simulink model "rfdc_awg"  (R2021a)
(part 2 of 30)

      mask prompts: io_names "Names [msb...lsb]"; io_widths "Bitwidths [msb...lsb]"; io_bps "Binary pts [msb...lsb]"; io_types "Data types [msb...lsb], ufix=0, fix=1, bool=2"; show_format "Print format string?"; snap_storage "Storage medium"; snap_dram_dimm "DRAM dimm"; snap_dram_clock "DRAM clock rate"; snap_nsamples "Number of Samples (2^?)"; snap_data_width "Data width"; snap_offset "Start delay support"; snap_circap "Circular capture support"; snap_value "Extra value capture support"; snap_ext_arm "External arm support"; snap_ext_circ "External circular capture support"; snap_provide_outputs "Provide outputs"; snap_use_dsp48 "Use DSP48s to implement counters"; snap_delay "Pre-snapshot delay"; extra_names "Names [msb...lsb]"; extra_widths "Widths [msb...lsb]"; extra_bps "Binary pts [msb...lsb]"; extra_types "Data types [msb...lsb], ufix=0, fix=1, bool=2"
      mask help:
      | A wrapped snapshot block. Allows specification of inputs to a snapblock word so the toolflow can automatically set up the scope.
      | See documentation for snapshot for explanation of parameters.
      mask init:
      | bitsnap_init(gcb);
      settings: AttributesFormatString=|
      | snap(1):uf128.0 = 128 bits\n128 wide, 16384 deep
      | debugID: 89627792
      mask TypeOptions snap_storage: bram | dram
      mask Callback snap_storage: bitsnap_callback();
      mask TypeOptions snap_dram_dimm: 1 | 2 | 3 | 4
      mask TypeOptions snap_dram_clock: 200 | 250 | 266 | 300 | 333
      mask TypeOptions snap_data_width: 8 | 16 | 32 | 64 | 128
      mask Callback snap_value: bitsnap_callback();
      mask Callback snap_ext_arm: bitsnap_callback();
      mask Callback snap_ext_circ: bitsnap_callback();
      mask Callback snap_provide_outputs: bitsnap_callback();
      mask DialogControl ParameterTabVar0 Prompt: Inputs
      mask DialogControl ParameterTabVar01 Prompt: Snapshot
      mask DialogControl ParameterTabVar012 Prompt: Extra Value
  snapshot_u2 : Subsystem  Tag=casper:bitsnap  AncestorBlock=casper_library_scopes/bitfield_snapshot  mask(bitsnap){io_names=[u2], io_widths=[128], io_bps=[0], io_types=[0], show_format=on, snap_storage=bram, snap_dram_dimm=2, snap_dram_clock=250, snap_nsamples=14, snap_data_width=128, snap_offset=off, snap_circap=off, snap_value=off, snap_ext_arm=off, snap_ext_circ=off, snap_provide_outputs=on, snap_use_dsp48=on, snap_delay=2, extra_names=[c d], extra_widths=[30 2], extra_bps=[0 0], extra_types=[0 0]}
      mask prompts: io_names "Names [msb...lsb]"; io_widths "Bitwidths [msb...lsb]"; io_bps "Binary pts [msb...lsb]"; io_types "Data types [msb...lsb], ufix=0, fix=1, bool=2"; show_format "Print format string?"; snap_storage "Storage medium"; snap_dram_dimm "DRAM dimm"; snap_dram_clock "DRAM clock rate"; snap_nsamples "Number of Samples (2^?)"; snap_data_width "Data width"; snap_offset "Start delay support"; snap_circap "Circular capture support"; snap_value "Extra value capture support"; snap_ext_arm "External arm support"; snap_ext_circ "External circular capture support"; snap_provide_outputs "Provide outputs"; snap_use_dsp48 "Use DSP48s to implement counters"; snap_delay "Pre-snapshot delay"; extra_names "Names [msb...lsb]"; extra_widths "Widths [msb...lsb]"; extra_bps "Binary pts [msb...lsb]"; extra_types "Data types [msb...lsb], ufix=0, fix=1, bool=2"
      mask help:
      | A wrapped snapshot block. Allows specification of inputs to a snapblock word so the toolflow can automatically set up the scope.
      | See documentation for snapshot for explanation of parameters.
      mask init:
      | bitsnap_init(gcb);
      settings: AttributesFormatString=|
      | snap(1):uf128.0 = 128 bits\n128 wide, 16384 deep
      | debugID: 89657583
      mask TypeOptions snap_storage: bram | dram
      mask Callback snap_storage: bitsnap_callback();
      mask TypeOptions snap_dram_dimm: 1 | 2 | 3 | 4
      mask TypeOptions snap_dram_clock: 200 | 250 | 266 | 300 | 333
      mask TypeOptions snap_data_width: 8 | 16 | 32 | 64 | 128
      mask Callback snap_value: bitsnap_callback();
      mask Callback snap_ext_arm: bitsnap_callback();
      mask Callback snap_ext_circ: bitsnap_callback();
      mask Callback snap_provide_outputs: bitsnap_callback();
      mask DialogControl ParameterTabVar0 Prompt: Inputs
      mask DialogControl ParameterTabVar01 Prompt: Snapshot
      mask DialogControl ParameterTabVar012 Prompt: Extra Value
  wires:
  Constant/1 -> snapshot_u1/2(we), snapshot_u2/2(we)
  edge_detect/1(out) -> snapshot_u1/3(trig), snapshot_u2/3(trig)
  snapshot_ctrl/1(in_start) -> edge_detect/1(in)
  Constant1/1 -> snapshot_ctrl/1(sim_1)
  Counter/1 -> Slice/1
  Slice/1 -> gpio/1
  gpio/1 -> Terminator/1
  ram_dac1/1(Out1) -> Concat3/1, snapshot_u1/1(in_u1)
  ram_dac1/2(Out2) -> Concat3/2, snapshot_u2/1(in_u2)
  ram_dac2/1(Out1) -> Concat1/1
  ram_dac2/2(Out2) -> Concat1/2
  ram_dac3/1(Out1) -> Concat2/1
  ram_dac3/2(Out2) -> Concat2/2
  ram_dac4/1(Out1) -> Concat4/1
  ram_dac4/2(Out2) -> Concat4/2
  ram_dac5/1(Out1) -> Concat5/1
  ram_dac5/2(Out2) -> Concat5/2
  ram_dac6/2(Out2) -> Concat6/2
  ram_dac6/1(Out1) -> Concat6/1
  ram_dac7/2(Out2) -> Concat7/2
  ram_dac7/1(Out1) -> Concat7/1
  ram_dac8/2(Out2) -> Concat8/2
  ram_dac8/1(Out1) -> Concat8/1
  ram_dac9/2(Out2) -> Concat9/2
  ram_dac9/1(Out1) -> Concat9/1
  ram_dac10/2(Out2) -> Concat10/2
  ram_dac10/1(Out1) -> Concat10/1
  ram_trig/1(Out1) -> Concat11/1
  ram_trig/2(Out2) -> Concat11/2
  Counter1/1 -> Relational/2, Scope/1, ram_trig/1(In1), ram_dac1/1(In1), ram_dac2/1(In1), ram_dac3/1(In1), ram_dac4/1(In1), ram_dac5/1(In1), ram_dac6/1(In1), ram_dac7/1(In1), ram_dac8/1(In1), ram_dac10/1(In1), ram_dac9/1(In1)
  Constant4/1 -> data_length/1(sim_1)
  data_length/1(in_reg) -> Relational/1
  Relational/1 -> Counter1/1
  Concat11/1 -> rfdc/2(s00_axis_tdata)
  Concat3/1 -> rfdc/3(s10_axis_tdata)
  Concat1/1 -> rfdc/4(s11_axis_tdata)
  Concat2/1 -> rfdc/5(s12_axis_tdata)
  Concat4/1 -> rfdc/6(s20_axis_tdata)
  Concat5/1 -> rfdc/7(s21_axis_tdata)
  Concat6/1 -> rfdc/8(s22_axis_tdata)
  Concat7/1 -> rfdc/9(s23_axis_tdata)
  Concat8/1 -> rfdc/10(s30_axis_tdata)
  Concat9/1 -> rfdc/11(s31_axis_tdata)
  Concat10/1 -> rfdc/12(s32_axis_tdata)
